simulink model "localizeAndControlUsingLidar"  (R2021b)
settings: Solver=VariableStepAuto  StartTime=0.0  StopTime=28.964  RelTol=1e-3
PreLoadFcn:
  | data = load('ReferencePathForward.mat');
  | 
  | refPosesX = data.ReferencePathForward.refPosesX;
  | refPosesY = data.ReferencePathForward.refPosesY;
  | refPosesT = data.ReferencePathForward.refPosesT;
  | 
  | if exist('lidarLocation','var') && exist('lidarOrientation','var')
  |     initPose = [lidarLocation(1,:) lidarOrientation(1, :)];
  | else
  |     initPose = [36.0913048  -9.4484911   1.6100000           0           0  -3.1311762];
  | end
  | 
  | helperSLCreateUtilityBus(1);
values from neighbouring files (symbols this model uses):
  centerToRear = 1.343    [LidarLocalizationInUnrealExample.m]
  curvatures = data.ReferencePathForward.Trajectory.curvatures    [LidarLocalizationInUnrealExample.m]
  directions = data.ReferencePathForward.Trajectory.directions    [LidarLocalizationInUnrealExample.m]
  refPoses = data.ReferencePathForward.Trajectory.refPoses    [LidarLocalizationInUnrealExample.m]
  startPose = refPoses(1, :)    [LidarLocalizationInUnrealExample.m]
  velocities = data.ReferencePathForward.Trajectory.velocities    [LidarLocalizationInUnrealExample.m]
libraries: drivingvehiclecontroller x2, simulink x2, simulink_extras x2, sim3dphyssensorlib x1, sim3dlib x1, sim3dautolib x1, autolibshared x1
settings Model: Creator=The MathWorks, Inc.  LastModifiedBy=The MathWorks, Inc.
settings SolverCC: AlgebraicLoopSolver=TrustRegion
settings DebuggingCC: SFMachineParentedDataDiag=warning

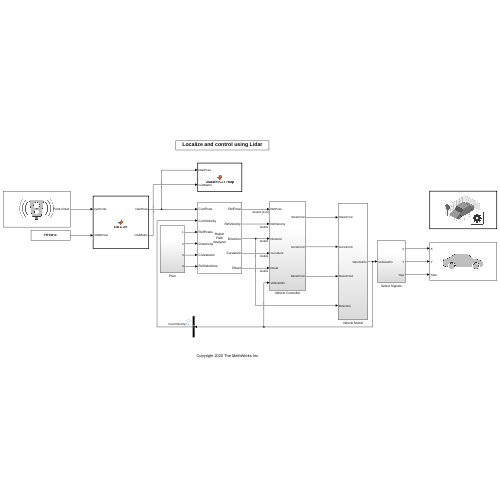
[thumbnail: Simulink's stored preview of the top-level diagram]
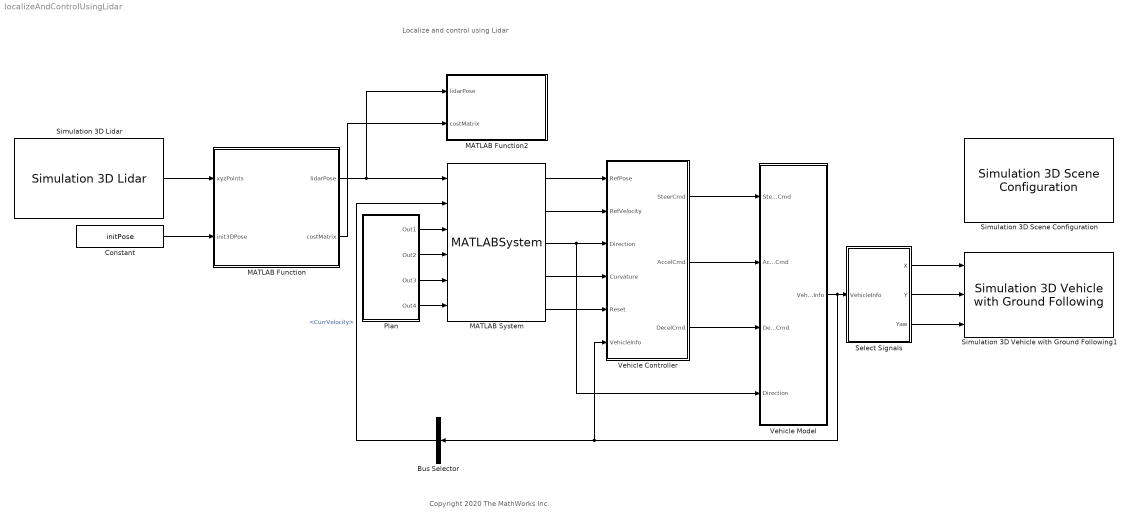
== system localizeAndControlUsingLidar ==
  note: Localize and control using Lidar
  note: Copyright 2020 The MathWorks Inc.
  Bus Selector : BusSelector  OutputSignals=CurrVelocity
  Constant : Constant  Value=initPose  VectorParams1D=off
  MATLAB Function : MATLAB Function  TreatAsAtomicUnit=on
  MATLAB Function2 : MATLAB Function  TreatAsAtomicUnit=on
      settings: ModelCloseFcn=|
      | hFigs = findobj(groot, 'Name', 'Costmap', 'Type', 'figure');
      | 
      | for n = 1 : numel(hFigs)
      |    hFig = hFigs(n);
      |    if isvalid(hFig)
      |       close(hFig);
      |    end
      | end
  MATLAB System : MATLABSystem  System=HelperPathAnalyzer  Wheelbase=2.6  HasResetOutput=on  SimulateUsing=Interpreted execution
      mask Type: HelperPathAnalyzer
      mask Display:
      | disp(['Helper' char(10) 'Path' char(10) 'Analyzer']);
      | port_label('input',1,'CurrPose');
      | port_label('input',2,'CurrVelocity');
      | port_label('input',3,'RefPoses');
      | port_label('input',4,'Directions');
      | port_label('input',5,'Curvatures');
      | port_label('input',6,'RefVelocities');
      | port_label('output',1,'RefPose');
      | port_label('output',2,'RefVelocity');
      | port_label('output',3,'Direction');
      | port_label('output',4,'Curvature');
      | port_label('output',5,'Reset');
  Plan : Subsystem
  Select Signals : Subsystem
  Simulation 3D Lidar : sim3dphyssensorlib/Simulation 3D Lidar  Priority=1  sensorTag=Sim3dSensor1  sensorId=1  sensorName=Sim3dSensor1  vehTagList={'Scene Origin';'SimulinkVehicle1'}  vehTag=SimulinkVehicle1  mountLoc=Roof center  offsetFlag=off  tmountOffset=[0, 0, 0]  rmountOffset=[0, 0, 0]  DetectionRange=90  RangeResolution=0.002  VerticalFOV=40  VerticalResolution=1.25  HorizontalFOV=360  HorizontalResolution=0.332409972299169  DistanceOutportEnabled=off  TransformOutportEnabled=off  SampleTime=0.1  mountPoint=[0 0 1.55999994277954]  mountOrientation=[0 0 0]  aMode=3  ID=1
      settings: SourceProductBaseCode=AE,DR,UV,VE
  Simulation 3D Scene Configuration : sim3dlib/Simulation 3D Scene Configuration  Priority=0  ProjectFormat_internal=Default Scenes  ProjectFormat=Default Scenes  SceneDesc=Large parking lot  ProjectName=/mathworks/devel/bat/BR2021bd/build/matlab/toolbox/shared/sim3d_projects/automotive_project/UE4/LinuxNoEditor/AutoVrtlEnv.sh  ScenePath=/Game/Maps/HwStrght  vehTagList={'Scene Origin';'SimulinkVehicle1'}  vehTag=SimulinkVehicle1  OpVisEn=off  Ts=0.02  EnableWindow=on  EnableWeather=off  SunAltitude=40.0  SunAzimuth=90  clouds=10  wind=1  fog=0  rain=0  sensorTag=MainCamera2  sensorId=2  sensorName=MainCamera2  mountLoc=Origin  offsetFlag=off  tmountOffset=[0, 0, 0]  rmountOffset=[0, 0, 0]  HorizontalResolution=1280  VerticalResolution=720  HorizontalFOV=60  mountPoint=[0 0 0]  mountOrientation=[0 0 0]  aMode=3  ID=2
      settings: SourceProductBaseCode=AE,DR,UV,VE
  Simulation 3D Vehicle with Ground Following1 : sim3dautolib/Simulation 3D Vehicle with Ground Following  Priority=-1  PassVehMesh=Hatchback  PassVehMesh_Internal=Muscle car  MeshPath=/MathWorksSimulation/Vehicles/Muscle/Meshes/SK_MuscleCar.SK_MuscleCar  TrackWidth=1.9  WheelBase=3  WheelRadius=0.35  VehColor=Red  VehColor_Internal=Red  InitialPos=[startPose(1)+cosd(startPose(3))*centerToRear, startPose(2)+sind(startPose(3))*centerToRear, 0]  InitialRot=[0, 0, startPose(3)]  ActorName=SimulinkVehicle1  SampleTime=0.02  ActorType=SimulinkVehicle  ID=1  aMode=3  ActorTag=SimulinkVehicle1  CoordinateScheme=ISO  VehLightsControl=off  HeadlightColor=[ 1, 1, 1 ]  HighBeamIntensity=100000  LowBeamIntensity=60000  HighBeamConeAngle=70  LowBeamConeAngle=70  LeftHeadlightOrientation=[ 0, 0 ]  RightHeadlightOrientation=[ 0, 0 ]  BrakelightIntensity=500  ReverselightIntensity=500  SignallightIntensity=500  SignallightPeriod=1  SignalPulseWidth=50  TransformOutportEnabled=off
      settings: SourceProductBaseCode=AE,DR,UV,VE
  Vehicle Controller : Subsystem
  Vehicle Model : Subsystem
  wires:
  Simulation 3D Lidar/1 -> MATLAB Function/1(xyzPoints)
  Constant/1 -> MATLAB Function/2(init3DPose)
  MATLAB Function/2(costMatrix) -> MATLAB Function2/2(costMatrix)
  MATLAB System/1 -> Vehicle Controller/1(RefPose)
  MATLAB System/2 -> Vehicle Controller/2(RefVelocity)
  MATLAB System/3 -> Vehicle Controller/3(Direction), Vehicle Model/4(Direction)
  MATLAB System/4 -> Vehicle Controller/4(Curvature)
  MATLAB System/5 -> Vehicle Controller/5(Reset)
  Vehicle Controller/1(SteerCmd) -> Vehicle Model/1(SteerCmd)
  Vehicle Controller/2(AccelCmd) -> Vehicle Model/2(AccelCmd)
  Vehicle Controller/3(DecelCmd) -> Vehicle Model/3(DecelCmd)
  Vehicle Model/1(VehicleInfo) -> Bus Selector/1, Vehicle Controller/6(VehicleInfo), Select Signals/1(VehicleInfo)
  Select Signals/1(X) -> Simulation 3D Vehicle with Ground Following1/1
  Select Signals/3(Yaw) -> Simulation 3D Vehicle with Ground Following1/3
  Select Signals/2(Y) -> Simulation 3D Vehicle with Ground Following1/2
  Bus Selector/1 -> MATLAB System/2  "<CurrVelocity>"
  MATLAB Function/1(lidarPose) -> MATLAB System/1, MATLAB Function2/1(lidarPose)
  Plan/1(Out1) -> MATLAB System/3
  Plan/2(Out2) -> MATLAB System/4
  Plan/3(Out3) -> MATLAB System/5
  Plan/4(Out4) -> MATLAB System/6

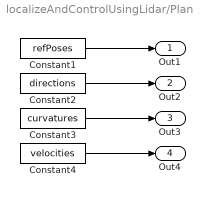
== system localizeAndControlUsingLidar/Plan ==
  Constant1 : Constant  Value=refPoses  VectorParams1D=off
  Constant2 : Constant  Value=directions
  Constant3 : Constant  Value=curvatures
  Constant4 : Constant  Value=velocities
  Out1 : Outport
  Out2 : Outport  Port=2
  Out3 : Outport  Port=3
  Out4 : Outport  Port=4
  wires:
  Constant2/1 -> Out2/1
  Constant3/1 -> Out3/1
  Constant4/1 -> Out4/1
  Constant1/1 -> Out1/1

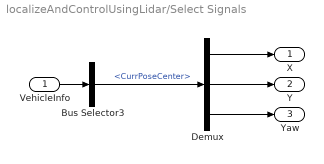
== system localizeAndControlUsingLidar/Select Signals ==
  VehicleInfo : Inport
  Bus Selector3 : BusSelector  OutputSignals=CurrPoseCenter
  Demux : Demux  Outputs=3
  X : Outport  VectorParamsAs1DForOutWhenUnconnected=off
  Y : Outport  Port=2  VectorParamsAs1DForOutWhenUnconnected=off
  Yaw : Outport  Port=3  VectorParamsAs1DForOutWhenUnconnected=off
  wires:
  Bus Selector3/1 -> Demux/1  "<CurrPoseCenter>"
  Demux/1 -> X/1
  VehicleInfo/1 -> Bus Selector3/1
  Demux/2 -> Y/1
  Demux/3 -> Yaw/1

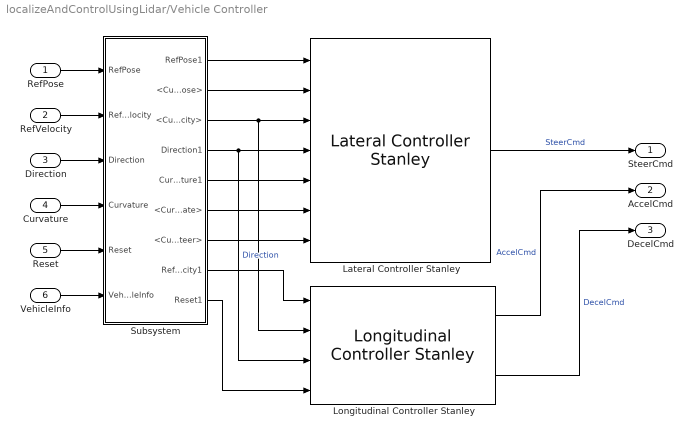
== system localizeAndControlUsingLidar/Vehicle Controller ==
  RefPose : Inport  OutDataTypeStr=double  PortDimensions=[1 3]  SampleTime=[0.050000000000000003,0]
  RefVelocity : Inport  Port=2  OutDataTypeStr=double  PortDimensions=[1 1]  SampleTime=[0.050000000000000003,0]
  Direction : Inport  Port=3  OutDataTypeStr=double  PortDimensions=[1 1]  SampleTime=[0.050000000000000003,0]
  Curvature : Inport  Port=4  OutDataTypeStr=double  PortDimensions=[1 1]  SampleTime=[0.050000000000000003,0]
  Reset : Inport  Port=5  OutDataTypeStr=double  PortDimensions=[1 1]  SampleTime=[0.050000000000000003,0]
  VehicleInfo : Inport  Port=6  OutDataTypeStr=Bus: vehicleInfoBus
  Lateral Controller Stanley : drivingvehiclecontroller/Lateral Controller Stanley  ModelType=Dynamic bicycle model  PositionGainF=3  PositionGainR=2.5  YawRateGain=0.25  DelayGain=0.2  VehicleMass=1575  Lf=1.104  Lr=1.343  TireStiffness=19000  Wheelbase=2.8  MaxSteeringAngle=45
      settings: SourceProductBaseCode=DR
  Longitudinal Controller Stanley : drivingvehiclecontroller/Longitudinal Controller Stanley  Kp=2.5  Ki=1  SampleTime=0.05  MaxAcceleration=3  MaxDeceleration=6
      settings: SourceProductBaseCode=DR
  Subsystem : Subsystem
  SteerCmd : Outport  VectorParamsAs1DForOutWhenUnconnected=off
  AccelCmd : Outport  Port=2  VectorParamsAs1DForOutWhenUnconnected=off
  DecelCmd : Outport  Port=3  VectorParamsAs1DForOutWhenUnconnected=off
  wires:
  RefPose/1 -> Subsystem/1(RefPose)
  Subsystem/3(<CurrVelocity>) -> Lateral Controller Stanley/3, Longitudinal Controller Stanley/2
  Longitudinal Controller Stanley/1 -> AccelCmd/1  "AccelCmd"
  Subsystem/9(Reset1) -> Longitudinal Controller Stanley/4
  VehicleInfo/1 -> Subsystem/6(VehicleInfo)
  RefVelocity/1 -> Subsystem/2(RefVelocity)
  Longitudinal Controller Stanley/2 -> DecelCmd/1  "DecelCmd"
  Direction/1 -> Subsystem/3(Direction)
  Subsystem/4(Direction1) -> Lateral Controller Stanley/4, Longitudinal Controller Stanley/3  "Direction"
  Subsystem/2(<CurrPose>) -> Lateral Controller Stanley/2
  Reset/1 -> Subsystem/5(Reset)
  Subsystem/8(RefVelocity1) -> Longitudinal Controller Stanley/1
  Subsystem/1(RefPose1) -> Lateral Controller Stanley/1
  Lateral Controller Stanley/1 -> SteerCmd/1  "SteerCmd"
  Curvature/1 -> Subsystem/4(Curvature)
  Subsystem/6(<CurrYawRate>) -> Lateral Controller Stanley/6
  Subsystem/5(Curvature1) -> Lateral Controller Stanley/5
  Subsystem/7(<CurrSteer>) -> Lateral Controller Stanley/7

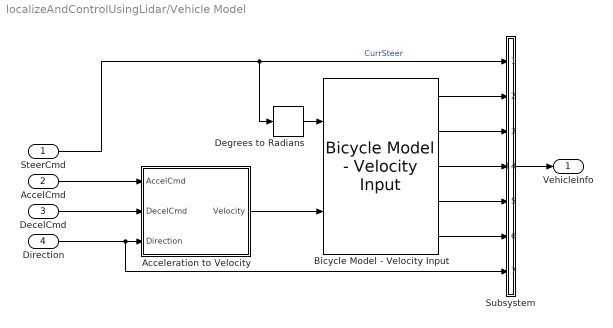
== system localizeAndControlUsingLidar/Vehicle Model ==
  SteerCmd : Inport
  AccelCmd : Inport  Port=2
  DecelCmd : Inport  Port=3
  Direction : Inport  Port=4
  Acceleration to Velocity : Subsystem  TreatAsAtomicUnit=on
  Bicycle Model - Velocity Input : autolibshared/Bicycle Model - Velocity Input  trackMode=Single (bicycle)  inputMode=External longitudinal forces  frontSteerMode=on  rearSteerMode=off  windMode=off  muMode=off  extFMode=off  extMMode=off  aMode=3  NF=2  NR=2  m=1575  a=centerToFront  b=centerToRear  h=0.227  X_o=startPose(1)+cosd(startPose(3))*centerToRear  xdot_o=0  CalphaMode=off  sigmaMode=on  w=[1.4,1.4]  Cy_f=19e3  Cy_r=20e3  sigma_f=.1  sigma_r=.1  alpha_f_brk=[-.1 .1]  Cy_f_data=[-9e3 9e3]  alpha_r_brk=[-.1 .1]  Cy_r_data=[-9e3 9e3]  Y_o=startPose(2) +sind(startPose(3))*centerToRear  ydot_o=0  Izz=4000  psi_o=deg2rad(startPose(3))  r_o=0  Af=2  Cd=.3  Cl=.1  Cpm=.1  beta_w=[0:0.01:0.3]  Cs=[0:0.03:0.9]  Cym=[0:0.01:0.3]  Pabs=101325  Tair=273  g=9.81  mu=1  xdot_tol=.01  Fznom=5000  Fxtire_sat=1e6  Fytire_sat=1e6  longOff=0  latOff=0  vertOff=0
      settings: SourceProductBaseCode=PW,DR,MT,UV,VE
  Degrees to Radians : simulink_extras/Transformations/Degrees to Radians
  Subsystem : Subsystem
  VehicleInfo : Outport  VectorParamsAs1DForOutWhenUnconnected=off
  wires:
  Acceleration to Velocity/1(Velocity) -> Bicycle Model - Velocity Input/2
  Direction/1 -> Subsystem/7(<Direction>), Acceleration to Velocity/3(Direction)
  Degrees to Radians/1 -> Bicycle Model - Velocity Input/1
  SteerCmd/1 -> Degrees to Radians/1, Subsystem/1(CurrSteer)  "CurrSteer"
  DecelCmd/1 -> Acceleration to Velocity/2(DecelCmd)
  AccelCmd/1 -> Acceleration to Velocity/1(AccelCmd)
  Subsystem/1(VehicleInfo) -> VehicleInfo/1
  Bicycle Model - Velocity Input/1 -> Subsystem/2(Info)
  Bicycle Model - Velocity Input/2 -> Subsystem/3(xdot)
  Bicycle Model - Velocity Input/3 -> Subsystem/4(ydot)
  Bicycle Model - Velocity Input/4 -> Subsystem/5(psi)
  Bicycle Model - Velocity Input/5 -> Subsystem/6(r)

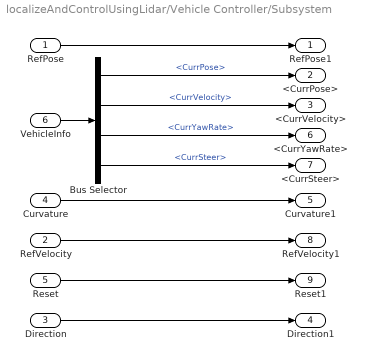
== system localizeAndControlUsingLidar/Vehicle Controller/Subsystem ==
  RefPose : Inport
  RefVelocity : Inport  Port=2
  Direction : Inport  Port=3
  Curvature : Inport  Port=4
  Reset : Inport  Port=5
  VehicleInfo : Inport  Port=6
  Bus Selector : BusSelector  OutputSignals=CurrPose,CurrVelocity,CurrYawRate,CurrSteer
  RefPose1 : Outport  VectorParamsAs1DForOutWhenUnconnected=off
  <CurrPose> : Outport  Port=2  VectorParamsAs1DForOutWhenUnconnected=off
  <CurrVelocity> : Outport  Port=3  VectorParamsAs1DForOutWhenUnconnected=off
  Direction1 : Outport  Port=4  VectorParamsAs1DForOutWhenUnconnected=off
  Curvature1 : Outport  Port=5  VectorParamsAs1DForOutWhenUnconnected=off
  <CurrYawRate> : Outport  Port=6  VectorParamsAs1DForOutWhenUnconnected=off
  <CurrSteer> : Outport  Port=7  VectorParamsAs1DForOutWhenUnconnected=off
  RefVelocity1 : Outport  Port=8  VectorParamsAs1DForOutWhenUnconnected=off
  Reset1 : Outport  Port=9  VectorParamsAs1DForOutWhenUnconnected=off
  wires:
  Bus Selector/4 -> <CurrSteer>/1  "<CurrSteer>"
  Curvature/1 -> Curvature1/1
  Bus Selector/3 -> <CurrYawRate>/1  "<CurrYawRate>"
  Reset/1 -> Reset1/1
  RefPose/1 -> RefPose1/1
  Bus Selector/1 -> <CurrPose>/1  "<CurrPose>"
  Bus Selector/2 -> <CurrVelocity>/1  "<CurrVelocity>"
  RefVelocity/1 -> RefVelocity1/1
  VehicleInfo/1 -> Bus Selector/1
  Direction/1 -> Direction1/1

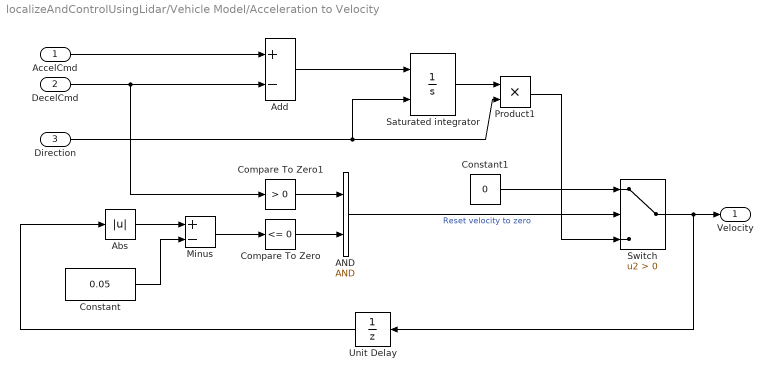
== system localizeAndControlUsingLidar/Vehicle Model/Acceleration to Velocity ==
  AccelCmd : Inport  PortDimensions=[1 1]
  DecelCmd : Inport  Port=2  PortDimensions=[1 1]
  Direction : Inport  Port=3
  AND : Logic  IconShape=distinctive  AllPortsSameDT=off  OutDataTypeStr=boolean
  Abs : Abs
  Add : Sum  Inputs=+-
  Compare To Zero : simulink/Logic and Bit Operations/Compare To Zero  relop=<=  OutDataTypeStr=boolean
  Compare To Zero1 : simulink/Logic and Bit Operations/Compare To Zero  relop=>  OutDataTypeStr=boolean
  Constant : Constant  Value=0.05
  Constant1 : Constant  Value=0
  Minus : Sum  Inputs=+-
  Product1 : Product
  Saturated integrator : Integrator  ExternalReset=either  LimitOutput=on  LowerSaturationLimit=0  AbsoluteTolerance=1e-3  ZeroCross=off
  Switch : Switch  Criteria=u2 > Threshold
  Unit Delay : UnitDelay  SampleTime=-1  HasFrameUpgradeWarning=on
  Velocity : Outport  VectorParamsAs1DForOutWhenUnconnected=off
  wires:
  Direction/1 -> Product1/2, Saturated integrator/2
  AccelCmd/1 -> Add/1
  Add/1 -> Saturated integrator/1
  DecelCmd/1 -> Compare To Zero1/1, Add/2
  Unit Delay/1 -> Abs/1
  Abs/1 -> Minus/1
  Constant/1 -> Minus/2
  Minus/1 -> Compare To Zero/1
  Compare To Zero/1 -> AND/2
  Compare To Zero1/1 -> AND/1
  AND/1 -> Switch/2  "Reset velocity to zero"
  Switch/1 -> Unit Delay/1, Velocity/1
  Constant1/1 -> Switch/1
  Saturated integrator/1 -> Product1/1
  Product1/1 -> Switch/3

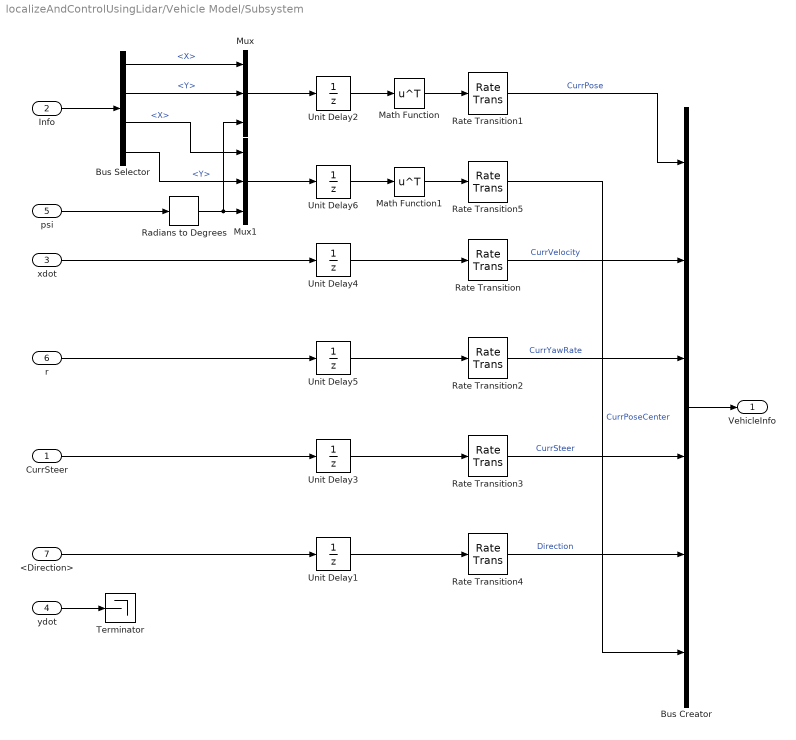
== system localizeAndControlUsingLidar/Vehicle Model/Subsystem ==
  CurrSteer : Inport
  Info : Inport  Port=2
  xdot : Inport  Port=3
  ydot : Inport  Port=4
  psi : Inport  Port=5
  r : Inport  Port=6
  <Direction> : Inport  Port=7
  Bus Creator : BusCreator  Inputs=6  OutDataTypeStr=Bus: vehicleInfoBus  NonVirtualBus=on
  Bus Selector : BusSelector  OutputSignals=InertFrm.RearAxl.Disp.X,InertFrm.RearAxl.Disp.Y,InertFrm.Cg.Disp.X,InertFrm.Cg.Disp.Y
  Math Function : Math  Operator=transpose  SignedPower=on  SaturateOnIntegerOverflow=on
  Math Function1 : Math  Operator=transpose  SignedPower=on  SaturateOnIntegerOverflow=on
  Mux : Mux  Inputs=3
  Mux1 : Mux  Inputs=3
  Radians to Degrees : simulink_extras/Transformations/Radians to Degrees
  Rate Transition : RateTransition  OutPortSampleTime=0.05
  Rate Transition1 : RateTransition  InitialCondition=startPose  OutPortSampleTime=0.05
  Rate Transition2 : RateTransition  OutPortSampleTime=0.05
  Rate Transition3 : RateTransition  OutPortSampleTime=0.05
  Rate Transition4 : RateTransition  InitialCondition=1  OutPortSampleTime=0.05
  Rate Transition5 : RateTransition  InitialCondition=[startPose(1)-cosd(startPose(3))*centerToRear,startPose(2)-sind(startPose(3))*centerToRear,startPose(3)]  OutPortSampleTime=0.05
  Terminator : Terminator
  Unit Delay1 : UnitDelay  InitialCondition=1  SampleTime=-1  HasFrameUpgradeWarning=on
  Unit Delay2 : UnitDelay  InitialCondition=startPose  SampleTime=-1  HasFrameUpgradeWarning=on
  Unit Delay3 : UnitDelay  SampleTime=-1  HasFrameUpgradeWarning=on
  Unit Delay4 : UnitDelay  SampleTime=-1  HasFrameUpgradeWarning=on
  Unit Delay5 : UnitDelay  SampleTime=-1  HasFrameUpgradeWarning=on
  Unit Delay6 : UnitDelay  InitialCondition=[startPose(1)-cosd(startPose(3))*centerToRear,startPose(2)-sind(startPose(3))*centerToRear,startPose(3)]  SampleTime=-1  HasFrameUpgradeWarning=on
  VehicleInfo : Outport  VectorParamsAs1DForOutWhenUnconnected=off
  wires:
  Unit Delay1/1 -> Rate Transition4/1
  CurrSteer/1 -> Unit Delay3/1
  Unit Delay5/1 -> Rate Transition2/1
  <Direction>/1 -> Unit Delay1/1
  Unit Delay4/1 -> Rate Transition/1
  Math Function/1 -> Rate Transition1/1
  Rate Transition/1 -> Bus Creator/2  "CurrVelocity"
  Unit Delay3/1 -> Rate Transition3/1
  Rate Transition3/1 -> Bus Creator/4  "CurrSteer"
  Rate Transition1/1 -> Bus Creator/1  "CurrPose"
  Rate Transition2/1 -> Bus Creator/3  "CurrYawRate"
  Rate Transition4/1 -> Bus Creator/5  "Direction"
  Unit Delay2/1 -> Math Function/1
  Info/1 -> Bus Selector/1
  Radians to Degrees/1 -> Mux1/3, Mux/3
  Bus Selector/2 -> Mux/2  "<Y>"
  Bus Selector/1 -> Mux/1  "<X>"
  Mux/1 -> Unit Delay2/1
  xdot/1 -> Unit Delay4/1
  ydot/1 -> Terminator/1
  r/1 -> Unit Delay5/1
  Bus Creator/1 -> VehicleInfo/1
  Bus Selector/4 -> Mux1/2  "<Y>"
  Mux1/1 -> Unit Delay6/1
  Unit Delay6/1 -> Math Function1/1
  Math Function1/1 -> Rate Transition5/1
  Rate Transition5/1 -> Bus Creator/6  "CurrPoseCenter"
  Bus Selector/3 -> Mux1/1  "<X>"
  psi/1 -> Radians to Degrees/1

== matlab function localizeAndControlUsingLidar/MATLAB Function ==
  data: xyzPoints input; lidarPose output; init3DPose input; costMatrix output
function [lidarPose, costMatrix] = Localize(xyzPoints, init3DPose)

coder.extrinsic('pointCloud', 'helperLidarRegistrationLocalizer', ...
    'localize', 'updateDisplay', 'rigid3d', 'helperExtract2DPose', 'struct', ...
    'helperPoseToRigidTransform', 'helperInterpolatePoseTform', 'createCostmap');

persistent frameCount lidarLocalizer relPoseTform currPoseTform isLocalizerActive prevCostmap;


mapSize       = [240 160];
spatialLimits = [0 60; -20 20; -Inf Inf];

if isempty(frameCount)
    frameCount = 0;
end

% Initialize lidarLocalizer
if isempty(lidarLocalizer)
    % Convert the pose to a rigid transformation object
    initTform = helperPoseToRigidTransform(init3DPose);
    
    % Rigid transformation object to convert from lidar sensor frame to
    % vehicle frame centered on the ground at the center of the rear-axle.
    % See https://www.mathworks.com/help/driving/ref/hatchback.html for
    % more details.
    lidarToVehicleTform = helperPoseToRigidTransform(single([0 0 -1.57 0 0 0]));
    
    % Specify display preferences
    displayPrefs = struct(...
        'View',                 '2D', ...                   % Display 2D top-view
        'VehicleDimensions',    [3.864, 1.960, 1.286], ...  % [length, width, height] of vehicle
        'VehicleColor',         [0.85 0.325 0.098], ...     % [R, G, B] color used to display vehicle
        'PoseOffset',           [0 0 -1.57], ...            % [x, y, z] offset to add to pose 
        'Limits',               [0 50 -25 10 -30 30], ...   % [xmin, xmax, ymin, ymax, zmin, zmax] map limits
        'Location',             'west');
    
    % Create a registration-based lidar localizer
    lidarLocalizer = helperLidarRegistrationLocalizer(...
        'InitialPoseTransform',     initTform, ...
        'LidarToVehicleTransform',  lidarToVehicleTform, ...
        'DisplayPreferences',       displayPrefs);
end

% Initialize poses
if isempty(currPoseTform)
    currPoseTform = rigid3d(eye(4,'single'));
end
if isempty(relPoseTform)
    relPoseTform = rigid3d(eye(4,'single'));
end
if isempty(isLocalizerActive)
    isLocalizerActive = false;
end

if isempty(prevCostmap)
    prevCostmap = ones(mapSize);
end

frameCount = frameCount + 1;

% Ignore first two frames
% Ignore point cloud with no valid points
hasNoPoints = all( isnan(xyzPoints), 'all' );
if hasNoPoints || frameCount < 2
    lidarPose = double(init3DPose([1 2 6]));
    
    costMatrix  = prevCostmap;
    return;
end

skipFrames = 5;
if mod(frameCount-1, skipFrames)==0
    isLocalizerActive = true;
    ptCloud = pointCloud(xyzPoints);
    
    [currPoseTform, relPoseTform] = localize(lidarLocalizer, ptCloud);
    
    updateDisplay(lidarLocalizer);
    drawnow update
    
    currPose = helperExtract2DPose(currPoseTform);
    
    % Convert to double and change radians to degrees
    lidarPose = double([currPose(1), currPose(2), rad2deg(currPose(3))]);
    
    costMatrix     = coder.nullcopy(ones(mapSize));
    costMatrix     = createCostmap(lidarLocalizer, mapSize, spatialLimits);
    prevCostmap = costMatrix;
else
    if ~isLocalizerActive
        lidarPose = double(init3DPose([1 2 6]));
        costMatrix  = prevCostmap;
        return;
    end
    
    % Interpolate between current pose transform and next pose transform,
    % i.e. assume constant velocity motion
    t = mod(frameCount-1, skipFrames)  / skipFrames;
    interpPoseTform = helperInterpolatePoseTform(currPoseTform, relPoseTform, t);
    
    currPose = helperExtract2DPose(interpPoseTform);
    
    % Convert to double and change radians to degrees
    lidarPose = double([currPose(1), currPose(2), rad2deg(currPose(3))]);
    costMatrix  = prevCostmap;
end

end

== matlab function localizeAndControlUsingLidar/MATLAB Function2 ==
  data: lidarPose input; costMatrix input
function VisualizeCostmap(lidarPose, costMatrix)

coder.extrinsic('inflationCollisionChecker', 'vehicleDimensions', 'get', ...
    'vehicleCostmap', 'fliplr', 'movegui', 'figure', 'plot', 'showShape');

persistent hAx hFig ccConfig
if isempty(hAx)
    hFig = figure('Name', 'Costmap');
    hAx = axes(hFig);
else
    hFig = get(hAx, 'Parent');
end

if isempty(ccConfig)
    % Specify vehicle dimensions
    % See https://www.mathworks.com/help/driving/ref/hatchback.html
    centerToFront = 1.104;
    centerToRear  = 1.343;
    frontOverhang = 0.828;
    rearOverhang  = 0.589;
    vehicleWidth  = 1.653;
    vehicleHeight = 1.513;
    vehicleLength = centerToFront + centerToRear + frontOverhang + rearOverhang;
    
    vehicleDims = vehicleDimensions(vehicleLength,vehicleWidth,vehicleHeight, ...
        'FrontOverhang',frontOverhang,'RearOverhang',rearOverhang);
    
    % Define collision-check configuration
    numCircles = 4;
    ccConfig = inflationCollisionChecker(vehicleDims, numCircles);
end

mapLocation = [0 -20];
cellSize    = 0.25; % in meters
costmap = vehicleCostmap(fliplr(costMatrix)', 'CellSize', cellSize, ...
    'MapLocation', mapLocation, 'CollisionChecker', ccConfig);

% Display the costmap
plot(costmap, 'Parent', hAx, 'Inflation', 'off');
movegui(hFig, 'east');

% Display current lidar pose
hold(hAx, 'on');
radius = 0.25;
showShape('circle', [lidarPose(1) lidarPose(2) radius], ...
    'Parent', hAx, 'Opacity', 1);
hold(hAx, 'off');    
end
